simulink model "aPegasusAutopilot"  (R2016a)
settings: Solver=ode4  StartTime=0.0  StopTime=inf  FixedStep=0.01  RelTol=1e-3
undefined symbols (not defined in the file or in its folder): Ue
libraries: xpcutilitieslib x2, instrumentlib x2, xpcobsoletelib x2
settings Model: PauseTimes=88  Creator=Marcelo Henrique  LastModifiedBy=Pegasus
settings DataIOCC: LimitDataPoints=on  SaveFormat=Array
settings DebuggingCC: AlgebraicLoopMsg=none  UnderspecifiedInitializationDetection=Classic  MergeDetectMultiDrivingBlocksExec=none  StateNameClashWarn=warning
settings HardwareCC: ProdBitPerPointer=32  ProdLargestAtomicFloat=None  ProdIntDivRoundTo=Undefined  ProdEndianess=Unspecified  ProdWordSize=32  ProdHWDeviceType=32-bit Generic
settings ModelReferenceCC: PropagateSignalLabelsOutOfModel=off
settings ConfigComp: CovModelRefEnable=Off

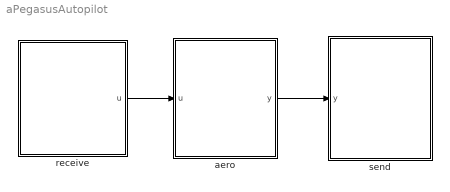
== system aPegasusAutopilot ==
  aero : Subsystem
  receive : Subsystem
  send : Subsystem
  wires:
  aero/1(y) -> send/1(y)
  receive/1(u) -> aero/1(u)

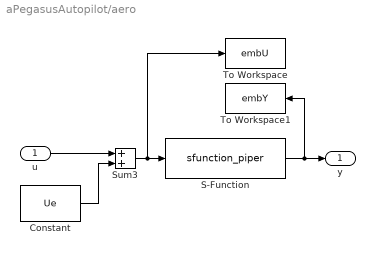
== system aPegasusAutopilot/aero ==
  u : Inport
  Constant : Constant  Value=Ue
  S-Function : S-Function  FunctionName=sfunction_piper  Parameters=par_gen,par_aero,par_prop, Xe  SFunctionDeploymentMode=off  EnableBusSupport=off
  Sum3 : Sum
  To Workspace : ToWorkspace  VariableName=embU  SaveFormat=Timeseries  SampleTime=-1
  To Workspace1 : ToWorkspace  VariableName=embY  SaveFormat=Timeseries  SampleTime=-1
  y : Outport
  wires:
  u/1 -> Sum3/1
  S-Function/1 -> To Workspace1/1, y/1
  Constant/1 -> Sum3/2
  Sum3/1 -> To Workspace/1, S-Function/1

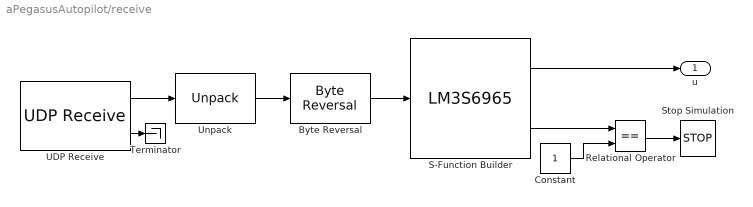
== system aPegasusAutopilot/receive ==
  Byte Reversal : xpcutilitieslib/Byte Reversal   numInp=1
  Constant : Constant
  Relational Operator : RelationalOperator  Operator===  OutDataTypeStr=boolean
  S-Function Builder : S-Function  InitFcn=try, set_param(gcb,'FunctionName','LM3S6965'), end  FunctionName=LM3S6965  SFunctionModules=LM3S6965_wrapper  SFunctionDeploymentMode=off  EnableBusSupport=off  mask(S-Function Builder){}
      mask help: Simulink:masks:SFunctionBuilder_MD
      mask init:
      | val = [[.9  0.75 0.75 1 1 .9 .9 1]',[1 1 0.75 0.75 .9 .9 1 .9]'];try , sys = get_param(gcb,'SfunBuilderFcnName');if isempty(sys), sys = get_param(gcb,'FunctionName'); end,catch, sys = get_param(gcb,'FunctionName'); end
      settings: CopyFcn=set_param(gcbh,'LinkStatus','none')  PreSaveFcn=try, set_param(gcb,'FunctionName','LM3S6965'), end  OpenFcn=sfunctionwizard(gcbh)
      mask Display: plot(val(:,1),val(:,2)),disp(sys), port_label('input',1,'Pkt'), port_label('output',1,'u'), port_label('output',2,'stop')
  Stop Simulation : Stop
  Terminator : Terminator
  UDP Receive : instrumentlib/UDP Receive  Host=192.168.1.101  Port=45004  LocalPort=45000  DataSize=23  EnableBlockingMode=off  Timeout=10  SampleTime=0.01  DataType=uint8  ByteOrder=BigEndian
  Unpack : xpcobsoletelib/Utilities/Unpack   dimensions={[1 23]}  datatypes={'uint8'}  byteAlign=1
  u : Outport
  wires:
  UDP Receive/1 -> Unpack/1
  Unpack/1 -> Byte Reversal/1
  UDP Receive/2 -> Terminator/1
  S-Function Builder/1 -> u/1
  Relational Operator/1 -> Stop Simulation/1
  Constant/1 -> Relational Operator/2
  Byte Reversal/1 -> S-Function Builder/1
  S-Function Builder/2 -> Relational Operator/1

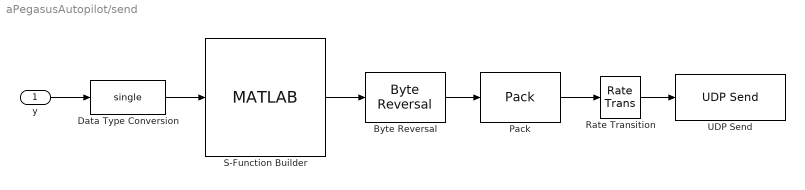
== system aPegasusAutopilot/send ==
  y : Inport
  Byte Reversal : xpcutilitieslib/Byte Reversal   numInp=1
  Data Type Conversion : DataTypeConversion  OutDataTypeStr=single
  Pack : xpcobsoletelib/Utilities/Pack   datatypes={'uint8'}  byteAlign=1
  Rate Transition : RateTransition  OutPortSampleTime=0.01
  S-Function Builder : S-Function  InitFcn=try, set_param(gcb,'FunctionName','MATLAB'), end  FunctionName=MATLAB  SFunctionModules=MATLAB_wrapper crc  SFunctionDeploymentMode=off  EnableBusSupport=off  mask(S-Function Builder){}
      mask help: Simulink:masks:SFunctionBuilder_MD
      mask init: same as aPegasusAutopilot/receive/S-Function Builder
      settings: CopyFcn=set_param(gcbh,'LinkStatus','none')  PreSaveFcn=try, set_param(gcb,'FunctionName','MATLAB'), end  OpenFcn=sfunctionwizard(gcbh)
      mask Display: plot(val(:,1),val(:,2)),disp(sys), port_label('input',1,'y'), port_label('output',1,'Pkt')
  UDP Send : instrumentlib/UDP Send  Host=192.168.1.101  Port=45004  LocalPort=45001  EnableBlockingMode=on  ByteOrder=BigEndian
  wires:
  Byte Reversal/1 -> Pack/1
  y/1 -> Data Type Conversion/1
  S-Function Builder/1 -> Byte Reversal/1
  Data Type Conversion/1 -> S-Function Builder/1
  Pack/1 -> Rate Transition/1
  Rate Transition/1 -> UDP Send/1
